simulink model "GMCLIB_SvmU0n_BAM"  (Simulink 8.3)
settings: Solver=ode45  StartTime=0.0  StopTime=10.0  RelTol=1e-3
settings Model: Creator=nxf41029  LastModifiedBy=nxf41029
settings DataIOCC: SignalLoggingSaveFormat=Dataset
settings DebuggingCC: UnderspecifiedInitializationDetection=Simplified  StateNameClashWarn=none
settings GRTTargetCC: CombineOutputUpdateFcns=on  GRTInterface=off

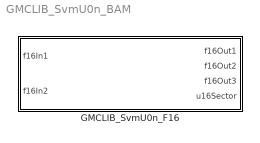
== system GMCLIB_SvmU0n_BAM ==
  GMCLIB_SvmU0n_F16 : Subsystem  mask(GMCLIB_SvmU0n_F16){}
      mask help: Bit accurate model of Standard Space Vector Modulation.
      mask init:
      | pos = get_param(gcb, 'Position');width = pos(3) - pos(1); height = pos(4) - pos(2);tX=width/2;tY=height*0.9;
      mask Display: color('black');port_label('input',1,'f16In1');port_label('input',2,'f16In2');port_label('output',1,'f16Out1');port_label('output',2,'f16Out2');port_label('output',3,'f16Out3');port_label('output',4,'u16Sector');color('black');disp('GMCLIB_SvmU0n_F16');color('blue');text(tX,tY, 'BAM', 'horizontalAlignment', 'center');

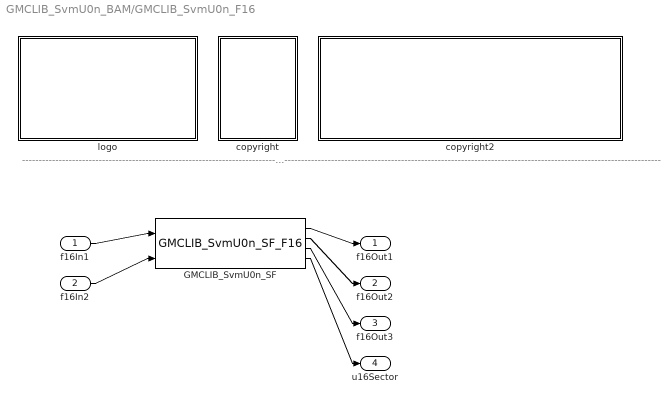
== system GMCLIB_SvmU0n_BAM/GMCLIB_SvmU0n_F16 ==
  note: ---------------------------------------------------------------------------------------------------------------------------------------------------------------------------------------------------
  f16In1 : Inport
  f16In2 : Inport  Port=2
  GMCLIB_SvmU0n_SF : S-Function  FunctionName=GMCLIB_SvmU0n_SF_F16  EnableBusSupport=off
  copyright : Subsystem
      mask Display: text(10,90,'FILE:');text(10,75,'DESRIPTION:');text(10,60,'COPYRIGHT:');text(10,45,'VERSION:');text(10,30,'DATE:')
  copyright2 : Subsystem
      mask Display: text(10,90,'GMCLIB_SvmU0n_BAM_F16.mdl');text(10,75,'Standard Space Vector Modulation.');text(10,60,'NXP');text(10,45,'0.1');text(10,30,'02-Apr-2019');
  logo : Subsystem
      mask Display: image(imread('logo.jpg'))
  f16Out1 : Outport
  f16Out2 : Outport  Port=2
  f16Out3 : Outport  Port=3
  u16Sector : Outport  Port=4
  wires:
  f16In1/1 -> GMCLIB_SvmU0n_SF/1
  f16In2/1 -> GMCLIB_SvmU0n_SF/2
  GMCLIB_SvmU0n_SF/1 -> f16Out1/1
  GMCLIB_SvmU0n_SF/2 -> f16Out2/1
  GMCLIB_SvmU0n_SF/3 -> f16Out3/1
  GMCLIB_SvmU0n_SF/4 -> u16Sector/1

== system GMCLIB_SvmU0n_BAM/GMCLIB_SvmU0n_F16/copyright ==

== system GMCLIB_SvmU0n_BAM/GMCLIB_SvmU0n_F16/copyright2 ==

== system GMCLIB_SvmU0n_BAM/GMCLIB_SvmU0n_F16/logo ==
